simulink model "rubik_cube_solver"  (R2022b)
settings: Solver=FixedStepDiscrete  StartTime=0.0  StopTime=10.0  RelTol=1e-3
InitFcn:
  | mbd_s32k_consistency_checks(bdroot(gcs));
undefined symbols (not defined in the file or in its folder): LQFP
libraries: mbd_s32k1xx_ec_toolbox x5
settings Model: Creator=leona  LastModifiedBy=aless
settings DataIOCC: ExternalInput=off  InitialState=off  SaveOutput=off  SignalLogging=off  SaveTime=off
settings OptimizationCC: DefaultParameterBehavior=Inlined  EnhancedBackFolding=on  PassReuseOutputArgsAs=Individual arguments  ZeroExternalMemoryAtStartup=off  ZeroInternalMemoryAtStartup=off  OptimizeBlockOrder=speed  DifferentSizesBufferReuse=on  OptimizationCustomize=off  EfficientTunableParamExpr=on
settings DebuggingCC: InheritedTsInSrcMsg=none  SingleTaskRateTransMsg=error  ParameterTunabilityLossMsg=error  UnconnectedInputMsg=error  UnconnectedOutputMsg=error  UnconnectedLineMsg=error  UnknownTsInhSupMsg=error
settings HardwareCC: ProdBitPerPointer=32  ProdBitPerSizeT=32  ProdBitPerPtrDiffT=32  ProdLargestAtomicInteger=Long  ProdLargestAtomicFloat=Double  ProdWordSize=32  ProdHWDeviceType=ARM Compatible->ARM Cortex
settings SFSimCC: MATLABDynamicMemAlloc=off
settings RTWCC: Description=Model Based Design Toolbox S32K1xx Code Generation Target  SystemTargetFile=mbd_s32k.tlc  MakeCommand=mbd_s32k_make_rtw COPY_MDLREF_INCLUDES=0  TemplateMakefile=mbd_s32k.tmf
settings CodeAppCC: ForceParamTrailComments=on  IgnoreCustomStorageClasses=off  OperatorAnnotations=on  SimulinkDataObjDesc=on  SFDataObjDesc=on  InsertBlockDesc=on
settings STFCustomTargetCC: TargetLangStandard=C99 (ISO)  MultiwordLength=256  CombineOutputUpdateFcns=on  ERTCustomFileBanners=on  SupportContinuousTime=off  SupportNonInlinedSFcns=off  RemoveResetFunc=on  MATLABClassNameForMDSCustomization=Simulink.SoftwareTarget.ERTCustomization  SystemTargetFile=mbd_s32k.tlc
settings ERTTargetCC: TargetLangStandard=C99 (ISO)  ParMdlRefBuildCompliant=off  CompOptLevelCompliant=off  ConcurrentExecutionCompliant=off  ModelStepFunctionPrototypeControlCompliant=off  CPPClassGenCompliant=off  UseToolchainInfoCompliant=off  InlinedParameterPlacement=NonHierarchical  ERTSrcFileBannerTemplate=mbd_ert_code_template.cgt  ERTHdrFileBannerTemplate=mbd_ert_code_template.cgt  ERTDataSrcFileTemplate=mbd_ert_code_template.cgt  ERTDataHdrFileTemplate=mbd_ert_code_template.cgt  ERTCustomFileTemplate=example_file_process.tlc

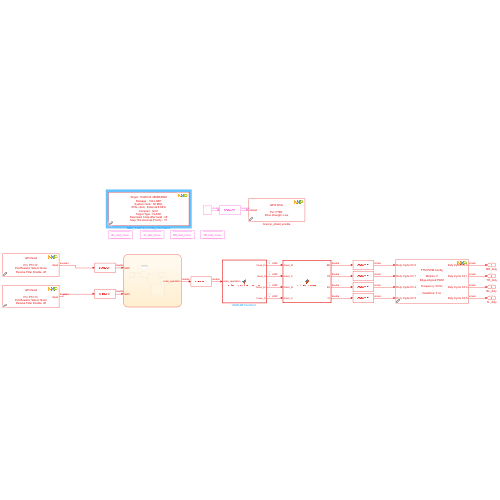
[thumbnail: Simulink's stored preview of the top-level diagram]
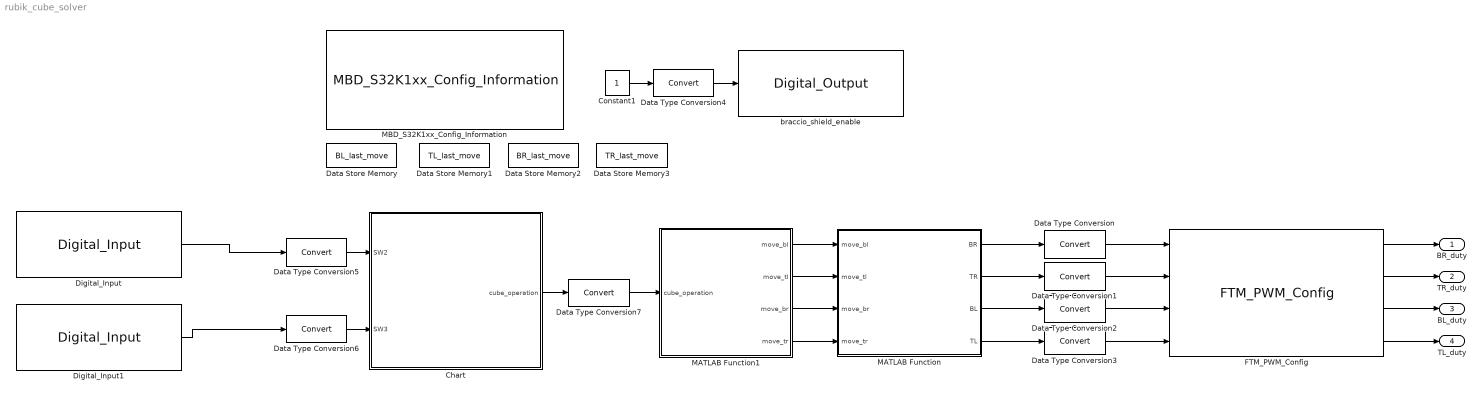
== system rubik_cube_solver ==
  Chart : Stateflow chart  TreatAsAtomicUnit=on
  Constant1 : Constant
  Data Store Memory : DataStoreMemory  DataStoreName=BL_last_move  WriteAfterWriteMsg=warning  ShowAdditionalParam=off
  Data Store Memory1 : DataStoreMemory  DataStoreName=TL_last_move  WriteAfterWriteMsg=warning  ShowAdditionalParam=off
  Data Store Memory2 : DataStoreMemory  DataStoreName=BR_last_move  WriteAfterWriteMsg=warning  ShowAdditionalParam=off
  Data Store Memory3 : DataStoreMemory  DataStoreName=TR_last_move  WriteAfterWriteMsg=warning  ShowAdditionalParam=off
  Data Type Conversion{,1..7} (8 alike) : DataTypeConversion  SaturateOnIntegerOverflow=off  RndMeth=Floor
  Digital_Input : mbd_s32k1xx_ec_toolbox/GPIO Blocks/Digital_Input  gpio_pin=PTC12: [PTC12 | Port C I/O]  pull_resistor=None  passive_filter=off
  Digital_Input1 : mbd_s32k1xx_ec_toolbox/GPIO Blocks/Digital_Input  gpio_pin=PTC13: [PTC13 | Port C I/O]  pull_resistor=None  passive_filter=off
  FTM_PWM_Config : mbd_s32k1xx_ec_toolbox/Motor Control Blocks/FTM Blocks/FTM_PWM_Config  ftmModule=0  ftmMode=Edge-Aligned PWM  ftmSourceClock=80 MHz  swcontrol_enable=off  chan0En=on  chan0Type=Independent  chan2En=off  chan2Type=Independent  chan4En=on  chan4Type=Independent  chan6En=off  chan6Type=Independent  ftmPwmUnits=Hz  outFrequency=50  ftmPeriod=25000  ftmPrescaler=Divide by 64  deadtimeUnits=Nanoseconds  deadtimeNs=0  deadtimeTicks=0  deadtimePrescaler=Divide by 1  dutyCycleCh0=0.03  dutyCycleCh1=0.125  dutyCycleCh2=0.025  dutyCycleCh3=0.025  dutyCycleCh4=0.025  dutyCycleCh5=0.025  dutyCycleCh6=0.25  dutyCycleCh7=0.25  dutyCycleSim=on  startAfterInit=on  showAdvOpt=on  pinFtmCh0=PTD15: [FTM0_CH0 | FTM Channel]  pinFtmCh1=PTD16: [FTM0_CH1 | FTM Channel]  pinPolCh0=Active High  pinPolCh1=Active High  outputComplem0=Main duplicated  outputLevel0=Low  outputLevel1=Low  pinFtmCh2=PTB14: [FTM0_CH2 | FTM Channel]  pinFtmCh3=PTC3: [FTM0_CH3 | FTM Channel]  pinPolCh2=Active High  pinPolCh3=Active High  outputComplem2=Main duplicated  outputLevel2=Low  outputLevel3=Low  pinFtmCh4=PTB4: [FTM0_CH4 | FTM Channel]  pinFtmCh5=PTB5: [FTM0_CH5 | FTM Channel]  pinPolCh4=Active High  pinPolCh5=Active High  outputComplem4=Main duplicated  outputLevel4=Low  outputLevel5=Low  pinFtmCh6=PTE8: [FTM0_CH6 | FTM Channel]  pinFtmCh7=None  pinPolCh6=Active High  pinPolCh7=Active High  outputComplem6=Main duplicated  outputLevel6=Low  outputLevel7=Low  initTrigger=off  chTrigger0=off  chTrigger1=off  chTrigger2=off  chTrigger3=off  chTrigger4=off  chTrigger5=off  chTrigger6=off  chTrigger7=off  mcuTargetUpdate=on  pwmSyncTrg=Software trigger  pwmSyncHwRouting=TRGMUX_FTM7  pwmSyncTrg0=off  pwmSyncTrg1=off  pwmSyncTrg2=off  pwmSyncAutoClear=on  pwmSyncMinLoad=on  pwmSyncMaxLoad=on  pwmSyncInvert=System Clock  pwmSyncOutControl=System Clock  pwmSyncOutMask=System Clock  pwmSyncCounterInitial=System Clock  pwmSyncPoints=Update now  reloadEnable=off  reloadPriority=15  reloadHalfCycle=off  reloadHCR=0  reloadFrequency=0  chnMatch0=off  chnMatch1=off  chnMatch2=off  chnMatch3=off  chnMatch4=off  chnMatch5=off  chnMatch6=off  chnMatch7=off  pwmFaultProtection=off  pwmFaultInterrupt=off  pwmFaultClearing=Fault control disabled  pwmFaultPinState=Safe Value  pwmFaultFilterValue=0  pwmFaultPriority=15  fault_disen_0=off  fault_filter_0=off  fault_polarity_0=Active High  fault_disen_1=off  fault_filter_1=off  fault_polarity_1=Active high  fault_disen_2=off  fault_filter_2=off  fault_polarity_2=Active high  fault_disen_3=off  fault_filter_3=off  fault_polarity_3=Active high  fault_pin_0=None  fault_pin_1=None  fault_pin_2=None  fault_pin_3=None
  MATLAB Function : MATLAB Function  TreatAsAtomicUnit=on
  MATLAB Function1 : MATLAB Function  TreatAsAtomicUnit=on
  MBD_S32K1xx_Config_Information : mbd_s32k1xx_ec_toolbox/MBD_S32K1xx_Config_Information  mbdt_ver=0  disp_str=|  config_params=[]  mcu_target_name=S32K144  mcu_target_package=100-LQFP  mcu_target_sram_size=48KB  mcu_system_clock_freq=80  mcu_xtal_freq=External 8  mcu_steptick_timer=LPIT Channel 0  mcu_steptick_prio=15  ds_import_enable=on  target_compiler=GCC  target_memory=FLASH  gcc_target_compile_opts=-mthumb -mfloat-abi=hard -mfpu=fpv4-sp-d16 -O1 -g -gstrict-dwarf  gcc_target_assemble_opts=-mthumb -mfloat-abi=hard -mfpu=fpv4-sp-d16 -g  gcc_target_link_opts=-mthumb -mfloat-abi=hard -mfpu=fpv4-sp-d16  gcc_target_default_lcf=on  gcc_target_user_lcf=S32K144_48_flash.ld  ghs_target_compile_opts=-cpu=cortexm4f -thumb -fpu=vfpv4_d16 -fsingle -Ogeneral -Wundef -Wimplicit-int -Wshadow -Wtrigraphs --no_commons --gnu_asm -gnu99 -gdwarf-2 -G  ghs_target_assemble_opts=-cpu=cortexm4f -fpu=vfpv4_d16  ghs_target_link_opts=-cpu=cortexm4f -thumb -fpu=vfpv4_d16  ghs_target_default_lcf=on  ghs_target_user_lcf=S32K144_48_flash.ld  iar_target_compile_opts=--cpu=Cortex-M4F --thumb --fpu=VFPv4_sp -Ol -e --debug --dlib_config normal  iar_target_assemble_opts=--cpu Cortex-M4F --thumb --fpu VFPv4_sp  iar_target_link_opts=--no_exceptions --vfe --inline  iar_target_default_lcf=on  iar_target_user_lcf=S32K144_48_flash.icf  pil_download_enable=off  rbl_download_enable=off  rbl_start_delay=5000  rbl_download_interface=OpenSDA  rbl_restart_request=off  rbl_com_port=Custom  rbl_com_port_custom=COM18  pil_download_rate=115200  pil_download_rate_custom=115200  pil_opensda_drive=Custom  pil_opensda_drive_custom=D  jtag_interface=OpenSDA Embedded Debug  jlink_default_path=on  jlink_user_path=C:\Program Files\SEGGER\JLink\  pil_uart_instance=1  pil_uart_rx=PTC6: [LPUART1_RX | Receive]  pil_uart_tx=PTC7: [LPUART1_TX | Transmit]  FTM_PWM_PcrCheckEnDis=on  FTM_Input_Edge_Inputs_PcrCheckEnDis=on  FTM_Dual_Edge_Inputs_PcrCheckEnDis=on  FTM_Quadrature_Inputs_PcrCheckEnDis=on  FTM_Hall_Sensor_Inputs_PcrCheckEnDis=on  LPTMR_PcrCheckEnDis=on  PIT_PcrCheckEnDis=on  RTC_PcrCheckEnDis=on  FlexCAN_PcrCheckEnDis=on  LIN_PcrCheckEnDis=on  FlexIO_PcrCheckEnDis=on  LPI2C_PcrCheckEnDis=on  LPSPI_PcrCheckEnDis=on  LPUART_PcrCheckEnDis=on  CMP_PcrCheckEnDis=on  GPIO_OutputPcrCheckEnDis=on  GPIO_InputPcrCheckEnDis=on  SBC_PcrCheckEnDis=on  BMS_PcrCheckEnDis=on  AMMCLIB_PcrCheckEnDis=on  FM_PcrCheckEnDis=on  Profile_PcrCheckEnDis=on  ConfigParams_PcrCheckEnDis=on  ModelRef_PcrCheckEnDis=on  PDB0_PcrCheckEnDis=on  CSEc_PcrCheckEnDis=on  eDMA_PcrCheckEnDis=on  FLASH_PcrCheckEnDis=on  ADC_PcrCheckEnDis=on  WDOG_PcrCheckEnDis=on
      | Target : S32K144-64KB_SRAM
      | Package : 100-pin
      | System clock : 80 MHz
      | XTAL clock : External 8 MHz
      | Compiler : IAR
      | Target Type : FLASH
      | Download Code after build : off
      | Step Tick Interrupt Priority : 15
  braccio_shield_enable : mbd_s32k1xx_ec_toolbox/GPIO Blocks/Digital_Output  gpio_pin=PTB3: [PTB3 | Port B I/O]  init_val=Low  drive_strength=Low
  BR_duty : Outport
  TR_duty : Outport  Port=2
  BL_duty : Outport  Port=3
  TL_duty : Outport  Port=4
  wires:
  Constant1/1 -> Data Type Conversion4/1
  Data Type Conversion1/1 -> FTM_PWM_Config/2
  Data Type Conversion3/1 -> FTM_PWM_Config/4
  MATLAB Function/2(TR) -> Data Type Conversion1/1
  FTM_PWM_Config/3 -> BL_duty/1
  FTM_PWM_Config/1 -> BR_duty/1
  Data Type Conversion/1 -> FTM_PWM_Config/1
  MATLAB Function1/2(move_tl) -> MATLAB Function/2(move_tl)
  FTM_PWM_Config/2 -> TR_duty/1
  Data Type Conversion2/1 -> FTM_PWM_Config/3
  FTM_PWM_Config/4 -> TL_duty/1
  MATLAB Function1/3(move_br) -> MATLAB Function/3(move_br)
  MATLAB Function1/4(move_tr) -> MATLAB Function/4(move_tr)
  MATLAB Function/4(TL) -> Data Type Conversion3/1
  MATLAB Function/1(BR) -> Data Type Conversion/1
  MATLAB Function/3(BL) -> Data Type Conversion2/1
  Data Type Conversion4/1 -> braccio_shield_enable/1
  MATLAB Function1/1(move_bl) -> MATLAB Function/1(move_bl)
  Data Type Conversion6/1 -> Chart/2(SW3)
  Data Type Conversion5/1 -> Chart/1(SW2)
  Digital_Input/1 -> Data Type Conversion5/1
  Digital_Input1/1 -> Data Type Conversion6/1
  Chart/1(cube_operation) -> Data Type Conversion7/1
  Data Type Conversion7/1 -> MATLAB Function1/1(cube_operation)

== matlab function rubik_cube_solver/MATLAB Function1 ==
  data: cube_operation input; move_bl output; move_tl output; move_br output; move_tr output
function [move_bl, move_tl, move_br, move_tr] = cube_operation_decoder(cube_operation)
% This function takes as input the code for a cube operation and converts
% it as positions of the 4 servo motors. The operations must be a 4 digit
% unsigned integer, encoded as follows:
%   - first digit [0, 1]: open/close left grip;
%   - second digit [0, 1]: open/close right grip;
%   - third digit [0, 1, 2]: set left arm to 90/0/180 degrees
%   - fourth digit [0, 1, 2]: set right arm to 90/0/180 degress

x1 = int32(mod(cube_operation/1000, 10));
x2 = int32(mod(cube_operation/100, 10));
x3 = int32(mod(cube_operation/10, 10));
x4 = int32(mod(cube_operation, 10));

move_tl = x1;
move_tr = x2;
move_bl = x3;
move_br = x4;

== matlab function rubik_cube_solver/MATLAB Function ==
  data: BR output; TR output; move_bl input; BL output; move_tl input; move_br input; move_tr input; TL output
function [BR, TR, BL, TL] = actuate_servos(move_bl, move_tl, move_br, move_tr)
% This function takes as input as specific number associated to a movement
% of the 4 servo motors (BL = Bottom Left, TL = Top Left, BR = Bottom Right,
% TR = Top Right) and it gives as output the 4 relative duty cycles needed to
% obtain that movement. 

min_duty = 0.025;
max_duty = 0.125;

duty_0_deg = min_duty;
duty_grip_open = min_duty + (max_duty-min_duty)/3;
duty_grip_closed = min_duty + (max_duty-min_duty)/15; 
duty_90_deg = min_duty + (max_duty-min_duty)/2;
duty_180_deg = max_duty;

switch (move_tl)
    case 0                  % Open left grip
        TL = duty_grip_open;
    case 1                  % Close left grip
        TL = duty_grip_closed;
    otherwise               % Open left grip
        TL = duty_grip_open;
end

switch (move_tr)
    case 0                  % Open right grip
        TR = duty_grip_open;
    case 1                  % Close right grip
        TR = duty_grip_closed;
    otherwise               % Open right grip
        TR = duty_grip_open;
end

switch (move_bl)
    case 0                  % Left arm straight
        BL = duty_90_deg;
    case 1                  % Left arm at 90° clockwise
        BL = duty_0_deg;
    case 2                 % Left arm at 90° counter-clockwise
        BL = duty_180_deg;
    otherwise
        BL = duty_90_deg;
end

switch (move_br)
    case 0                  % Right arm straight
        BR = duty_90_deg;
    case 1                  % Right arm at 90° clockwise
        BR = duty_0_deg;
    case 2                 % Right arm at 90° counter-clockwise
        BR = duty_180_deg;
    otherwise
        BR = duty_90_deg;
end

% Update current position of the motors
BL_last_move = move_bl;
TL_last_move = move_tl;
BR_last_move = move_br;
TR_last_move = move_tr;

== stateflow chart rubik_cube_solver/Chart ==
  state Li [commented out]
    en:
    %LTpp
    %RMm
    state fase1 [commented out]
      en:
      cube_operation=0100;
    state fase1bis [commented out]
      en:
      cube_operation=0110;
    state fase2 [commented out]
      en:
      cube_operation=1110;
    state fase4 [commented out]
      en:
      cube_operation=1120;
    state fase3bis [commented out]
      en:
      cube_operation=1020;
    state fase3 [commented out]
      en:
      cube_operation=1010;
    state fase5bis [commented out]
      en:
      cube_operation=0100;
    state fase6 [commented out]
      en:
      cube_operation=1100
    state fase5 [commented out]
      en:
      cube_operation=0120;
    state fase8bis [commented out]
      en:
      cube_operation=1000;
    state fase8 [commented out]
      en:
      cube_operation=1001;
    state fase7 %RMm [commented out]
      en:
      cube_operation=1101;
    state fase9 [commented out]
      en:
      cube_operation=1100;
    (default) -> Li.fase1 [commented out]
    Li.fase1 -> Li.fase1bis [commented out] : [after(delay_ms,msec)]
    Li.fase1bis -> Li.fase2 [commented out] : [after(delay_ms,msec)]
    Li.fase2 -> Li.fase3 [commented out] : [after(delay_ms,msec)]
    Li.fase3bis -> Li.fase4 [commented out] : [after(delay_ms,msec)]
    Li.fase3 -> Li.fase3bis [commented out] : [after(delay_ms,msec)]
    Li.fase4 -> Li.fase5 [commented out] : [after(delay_ms,msec)]
    Li.fase5bis -> Li.fase6 [commented out] : [after(delay_ms,msec)]
    Li.fase5 -> Li.fase5bis [commented out] : [after(delay_ms,msec)]
    Li.fase6 -> fase7 %RMm [commented out] : [after(delay_ms,msec)]
    fase7 %RMm -> Li.fase8 [commented out] : [after(delay_ms,msec)]
    Li.fase8 -> fase8bis [commented out] : [after(delay_ms,msec)]
    fase8bis -> Li.fase9 [commented out] : [after(delay_ms,msec)]
  state L [commented out]
    en:
    %LTpp
    %RMp
    state fase1 [commented out]
      en:
      cube_operation=0100;
    state fase1bis [commented out]
      en:
      cube_operation=0110;
    state fase2 [commented out]
      en:
      cube_operation=1110;
    state fase4 [commented out]
      en:
      cube_operation=1120;
    state fase3bis [commented out]
      en:
      cube_operation=1020;
    state fase3 [commented out]
      en:
      cube_operation=1010;
    state fase5bis [commented out]
      en:
      cube_operation=0100;
    state fase6 [commented out]
      en:
      cube_operation=1100
    state fase5 [commented out]
      en:
      cube_operation=0120;
    state fase8 [commented out]
      en:
      cube_operation=1101;
    state fase7bis [commented out]
      en:
      cube_operation=1001;
    state fase7 %RMp [commented out]
      en:
      cube_operation=1000;
    state fase9 [commented out]
      en:
      cube_operation=1100;
    L.fase1 -> L.fase1bis [commented out] : [after(delay_ms,msec)]
    L.fase1bis -> L.fase2 [commented out] : [after(delay_ms,msec)]
    L.fase2 -> L.fase3 [commented out] : [after(delay_ms,msec)]
    L.fase3bis -> L.fase4 [commented out] : [after(delay_ms,msec)]
    L.fase3 -> L.fase3bis [commented out] : [after(delay_ms,msec)]
    L.fase4 -> L.fase5 [commented out] : [after(delay_ms,msec)]
    L.fase5bis -> L.fase6 [commented out] : [after(delay_ms,msec)]
    L.fase5 -> L.fase5bis [commented out] : [after(delay_ms,msec)]
    L.fase6 -> fase7 %RMp [commented out] : [after(delay_ms,msec)]
    fase7 %RMp -> L.fase7bis [commented out] : [after(delay_ms,msec)]
    L.fase7bis -> L.fase8 [commented out] : [after(delay_ms,msec)]
    L.fase8 -> L.fase9 [commented out] : [after(delay_ms,msec)]
  state L2 [commented out]
    en:
    %LTpp
    %RMpp
    state fase1 [commented out]
      en:
      cube_operation=0100;
    state fase1bis [commented out]
      en:
      cube_operation=0110;
    state fase2 [commented out]
      en:
      cube_operation=1110;
    state fase4 [commented out]
      en:
      cube_operation=1120;
    state fase3bis [commented out]
      en:
      cube_operation=1020;
    state fase3 [commented out]
      en:
      cube_operation=1010;
    state fase5bis [commented out]
      en:
      cube_operation=0100;
    state fase6 [commented out]
      en:
      cube_operation=1100
    state fase5 [commented out]
      en:
      cube_operation=0120;
    state fase12 %RMpp [commented out]
      en:
      cube_operation=1000;
    state fase7bis [commented out]
      en:
      cube_operation=1001;
    state fase9 [commented out]
      en:
      cube_operation=1102;
    state fase8 [commented out]
      en:
      cube_operation=1101;
    state fase10 [commented out]
      en:
      cube_operation=1002;
    state fase11 [commented out]
      en:
      cube_operation=1100;
    state fase10bis [commented out]
      en:
      cube_operation=1000;
    L2.fase1 -> L2.fase1bis [commented out] : [after(delay_ms,msec)]
    L2.fase1bis -> L2.fase2 [commented out] : [after(delay_ms,msec)]
    L2.fase2 -> L2.fase3 [commented out] : [after(delay_ms,msec)]
    L2.fase3bis -> L2.fase4 [commented out] : [after(delay_ms,msec)]
    L2.fase3 -> L2.fase3bis [commented out] : [after(delay_ms,msec)]
    L2.fase4 -> L2.fase5 [commented out] : [after(delay_ms,msec)]
    L2.fase5bis -> L2.fase6 [commented out] : [after(delay_ms,msec)]
    L2.fase5 -> L2.fase5bis [commented out] : [after(delay_ms,msec)]
    L2.fase6 -> fase12 %RMpp [commented out] : [after(delay_ms,msec)]
    fase12 %RMpp -> L2.fase7bis [commented out] : [after(delay_ms,msec)]
    L2.fase7bis -> L2.fase8 [commented out] : [after(delay_ms,msec)]
    L2.fase9 -> L2.fase10 [commented out] : [after(delay_ms,msec)]
    L2.fase8 -> L2.fase9 [commented out] : [after(delay_ms,msec)]
    L2.fase10 -> fase10bis [commented out] : [after(delay_ms,msec)]
    fase10bis -> L2.fase11 [commented out] : [after(delay_ms,msec)]
  state U [commented out]
    %RTpp
    %LMp
    state fase1 %RTpp [commented out]
      en:
      cube_operation=1000;
    state fase2 [commented out]
      en:
      cube_operation=1001;
    state fase3 [commented out]
      en:
      cube_operation=1101;
    state fase6 [commented out]
      en:
      cube_operation=1102;
    state fase5 [commented out]
      en:
      cube_operation=0102;
    state fase4 [commented out]
      en:
      cube_operation=0101;
    state fase8 [commented out]
      en:
      cube_operation=1000;
    state fase9 [commented out]
      en:
      cube_operation=1100;
    state fase7 [commented out]
      en:
      cube_operation=1002;
    state fase12 [commented out]
      en:
      cube_operation=1110;
    state fase11 [commented out]
      en:
      cube_operation=0110;
    state fase10 %LMp [commented out]
      en:
      cube_operation=0100;
    state fase13 [commented out]
      en:
      cube_operation=1100;
    (default) -> U.fase1 %RTpp [commented out]
    U.fase2 -> U.fase3 [commented out] : [after(delay_ms,msec)]
    U.fase1 %RTpp -> U.fase2 [commented out] : [after(delay_ms,msec)]
    U.fase3 -> U.fase4 [commented out] : [after(delay_ms,msec)]
    U.fase4 -> U.fase5 [commented out] : [after(delay_ms,msec)]
    U.fase5 -> U.fase6 [commented out] : [after(delay_ms,msec)]
    U.fase6 -> U.fase7 [commented out] : [after(delay_ms,msec)]
    U.fase7 -> U.fase8 [commented out] : [after(delay_ms,msec)]
    U.fase8 -> U.fase9 [commented out] : [after(delay_ms,msec)]
    U.fase9 -> fase10 %LMp [commented out] : [after(delay_ms,msec)]
    U.fase11 -> U.fase12 [commented out] : [after(delay_ms,msec)]
    fase10 %LMp -> U.fase11 [commented out] : [after(delay_ms,msec)]
    U.fase12 -> U.fase13 [commented out] : [after(delay_ms,msec)]
  state U2 [commented out]
    %RTpp
    %LMpp
    state fase1 %RTpp [commented out]
      en:
      cube_operation=1000;
    state fase2 [commented out]
      en:
      cube_operation=1001;
    state fase3 [commented out]
      en:
      cube_operation=1101;
    state fase6 [commented out]
      en:
      cube_operation=1102;
    state fase5 [commented out]
      en:
      cube_operation=0102;
    state fase4 [commented out]
      en:
      cube_operation=0101;
    state fase8 [commented out]
      en:
      cube_operation=1000;
    state fase9 [commented out]
      en:
      cube_operation=1100;
    state fase7 [commented out]
      en:
      cube_operation=1002;
    state fase11 [commented out]
      en:
      cube_operation=0110;
    state fase10 %LMpp [commented out]
      en:
      cube_operation=0100;
    state fase12 [commented out]
      en:
      cube_operation=1110;
    state fase13 [commented out]
      en:
      cube_operation=1120;
    state fase14 [commented out]
      en:
      cube_operation=0120;
    state fase15 [commented out]
      en:
      cube_operation=0100;
    state fase16 [commented out]
      en:
      cube_operation=1100;
    (default) -> U2.fase1 %RTpp [commented out]
    U2.fase2 -> U2.fase3 [commented out] : [after(delay_ms,msec)]
    U2.fase1 %RTpp -> U2.fase2 [commented out] : [after(delay_ms,msec)]
    U2.fase3 -> U2.fase4 [commented out] : [after(delay_ms,msec)]
    U2.fase4 -> U2.fase5 [commented out] : [after(delay_ms,msec)]
    U2.fase5 -> U2.fase6 [commented out] : [after(delay_ms,msec)]
    U2.fase6 -> U2.fase7 [commented out] : [after(delay_ms,msec)]
    U2.fase7 -> U2.fase8 [commented out] : [after(delay_ms,msec)]
    U2.fase8 -> U2.fase9 [commented out] : [after(delay_ms,msec)]
    U2.fase9 -> fase10 %LMpp [commented out] : [after(delay_ms,msec)]
    U2.fase11 -> U2.fase12 [commented out] : [after(delay_ms,msec)]
    fase10 %LMpp -> U2.fase11 [commented out] : [after(delay_ms,msec)]
    U2.fase12 -> U2.fase13 [commented out] : [after(delay_ms,msec)]
    U2.fase13 -> fase14 [commented out] : [after(delay_ms,msec)]
    fase14 -> fase15 [commented out] : [after(delay_ms,msec)]
    fase15 -> fase16 [commented out] : [after(delay_ms,msec)]
  state waiting_for_cube
    en:
    %R = randi([1, 6], 3, 3, 6);
    solution = string(repmat(' ', 1, 45))
    %sol=Solve45(rubgen(3,23))
    sequence
    du:
    cube_operation=0100;
    SW2_status=SW2;
    end
  state waiting_to_start
    en:
    du:
    cube_operation=1100;
    SW2_status=SW2;
    SW3_status=SW3;
  state cube_reading
    en:
  state cube_solving
    en:
  state Ui [commented out]
    %RTpp
    %LMm
    state fase1 %RTpp [commented out]
      en:
      cube_operation=1000;
    state fase2 [commented out]
      en:
      cube_operation=1001;
    state fase3 [commented out]
      en:
      cube_operation=1101;
    state fase6 [commented out]
      en:
      cube_operation=1102;
    state fase5 [commented out]
      en:
      cube_operation=0102;
    state fase4 [commented out]
      en:
      cube_operation=0101;
    state fase8 [commented out]
      en:
      cube_operation=1000;
    state fase9 [commented out]
      en:
      cube_operation=1100;
    state fase7 [commented out]
      en:
      cube_operation=1002;
    state fase12 [commented out]
      en:
      cube_operation=0100;
    state fase11 [commented out]
      en:
      cube_operation=0110;
    state fase10 %LMm [commented out]
      en:
      cube_operation=1110;
    state fase13 [commented out]
      en:
      cube_operation=1100;
    (default) -> Ui.fase1 %RTpp [commented out]
    Ui.fase2 -> Ui.fase3 [commented out] : [after(delay_ms,msec)]
    Ui.fase1 %RTpp -> Ui.fase2 [commented out] : [after(delay_ms,msec)]
    Ui.fase3 -> Ui.fase4 [commented out] : [after(delay_ms,msec)]
    Ui.fase4 -> Ui.fase5 [commented out] : [after(delay_ms,msec)]
    Ui.fase5 -> Ui.fase6 [commented out] : [after(delay_ms,msec)]
    Ui.fase6 -> Ui.fase7 [commented out] : [after(delay_ms,msec)]
    Ui.fase7 -> Ui.fase8 [commented out] : [after(delay_ms,msec)]
    Ui.fase8 -> Ui.fase9 [commented out] : [after(delay_ms,msec)]
    Ui.fase9 -> fase10 %LMm [commented out] : [after(delay_ms,msec)]
    Ui.fase11 -> Ui.fase12 [commented out] : [after(delay_ms,msec)]
    fase10 %LMm -> Ui.fase11 [commented out] : [after(delay_ms,msec)]
    Ui.fase12 -> Ui.fase13 [commented out] : [after(delay_ms,msec)]
  state F [commented out]
    en:
    %RTm
    %LMp
    state fase1 [commented out]
      en:
      cube_operation=0100;
    state fase2 [commented out]
      en:
      cube_operation=0101;
    state fase3 [commented out]
      en:
      cube_operation=1101;
    state fase6 [commented out]
      en:
      cube_operation=1100
    state fase5 [commented out]
      en:
      cube_operation=1000;
    state fase4 [commented out]
      en:
      cube_operation=1001;
    state fase7 %LMp [commented out]
      en:
      cube_operation=0100;
    state fase8 [commented out]
      en:
      cube_operation=0110;
    state fase9 [commented out]
      en:
      cube_operation=1110;
    state fase10 [commented out]
      en:
      cube_operation=1100;
    (default) -> F.fase1 [commented out]
    F.fase2 -> F.fase3 [commented out] : [after(delay_ms,msec)]
    F.fase1 -> F.fase2 [commented out] : [after(delay_ms,msec)]
    F.fase3 -> F.fase4 [commented out] : [after(delay_ms,msec)]
    F.fase5 -> F.fase6 [commented out] : [after(delay_ms,msec)]
    F.fase4 -> F.fase5 [commented out] : [after(delay_ms,msec)]
    F.fase6 -> F.fase7 %LMp [commented out] : [after(delay_ms,msec)]
    F.fase7 %LMp -> F.fase8 [commented out] : [after(delay_ms,msec)]
    F.fase9 -> F.fase10 [commented out] : [after(delay_ms,msec)]
    F.fase8 -> F.fase9 [commented out] : [after(delay_ms,msec)]
  state Di [commented out]
    en:
    %LMm
    state fase1 %LMm [commented out]
      en:
      cube_operation=1110;
    state fase2 [commented out]
      en:
      cube_operation=0110;
    state fase3 [commented out]
      en:
      cube_operation=0100;
    state fase4 [commented out]
      en:
      cube_operation=1100;
    (default) -> fase1 %LMm [commented out]
    fase1 %LMm -> Di.fase2 [commented out] : [after(delay_ms,msec)]
    Di.fase2 -> Di.fase3 [commented out] : [after(delay_ms,msec)]
    Di.fase3 -> Di.fase4 [commented out] : [after(delay_ms,msec)]
  state R [commented out]
    en:
    %RMp
    state fase1 %RMp [commented out]
      en:
      cube_operation=1000;
    state fase2 [commented out]
      en:
      cube_operation=1001;
    state fase3 [commented out]
      en:
      cube_operation=1101;
    state fase4 [commented out]
      en:
      cube_operation=1100;
    (default) -> fase1 %RMp [commented out]
    fase1 %RMp -> R.fase2 [commented out] : [after(delay_ms,msec)]
    R.fase2 -> R.fase3 [commented out] : [after(delay_ms,msec)]
    R.fase3 -> R.fase4 [commented out] : [after(delay_ms,msec)]
  state R2 [commented out]
    en:
    %RMpp
    state fase1 %RMpp [commented out]
      en:
      cube_operation=1000;
    state fase2 [commented out]
      en:
      cube_operation=1001;
    state fase4 [commented out]
      en:
      cube_operation=1102;
    state fase3 [commented out]
      en:
      cube_operation=1101;
    state fase5 [commented out]
      en:
      cube_operation=1002;
    state fase6 [commented out]
      en:
      cube_operation=1000;
    state fase7 [commented out]
      en:
      cube_operation=1100;
    (default) -> fase1 %RMpp [commented out]
    fase1 %RMpp -> R2.fase2 [commented out] : [after(delay_ms,msec)]
    R2.fase2 -> R2.fase3 [commented out] : [after(delay_ms,msec)]
    R2.fase3 -> R2.fase4 [commented out] : [after(delay_ms,msec)]
    R2.fase4 -> R2.fase5 [commented out] : [after(delay_ms,msec)]
    R2.fase5 -> R2.fase6 [commented out] : [after(delay_ms,msec)]
    R2.fase6 -> R2.fase7 [commented out] : [after(delay_ms,msec)]
  state D [commented out]
    en:
    %LMp
    state fase1 %LMp [commented out]
      en:
      cube_operation=0100;
    state fase2 [commented out]
      en:
      cube_operation=0110;
    state fase3 [commented out]
      en:
      cube_operation=1110;
    state fase4 [commented out]
      en:
      cube_operation=1100;
    (default) -> fase1 %LMp [commented out]
    fase1 %LMp -> D.fase2 [commented out] : [after(delay_ms,msec)]
    D.fase2 -> D.fase3 [commented out] : [after(delay_ms,msec)]
    D.fase3 -> D.fase4 [commented out] : [after(delay_ms,msec)]
  state D2 [commented out]
    en:
    %LMpp
    state fase1 %LMpp [commented out]
      en:
      cube_operation=0100;
    state fase2 [commented out]
      en:
      cube_operation=0110;
    state fase4 [commented out]
      en:
      cube_operation=1120;
    state fase3 [commented out]
      en:
      cube_operation=1110;
    state fase6 [commented out]
      en:
      cube_operation=0100;
    state fase5 [commented out]
      en:
      cube_operation=0120;
    state fase7 [commented out]
      en:
      cube_operation=1100;
    (default) -> fase1 %LMpp [commented out]
    fase1 %LMpp -> D2.fase2 [commented out] : [after(delay_ms,msec)]
    D2.fase2 -> D2.fase3 [commented out] : [after(delay_ms,msec)]
    D2.fase3 -> D2.fase4 [commented out] : [after(delay_ms,msec)]
    D2.fase4 -> D2.fase5 [commented out] : [after(delay_ms,msec)]
    D2.fase5 -> D2.fase6 [commented out] : [after(delay_ms,msec)]
    D2.fase6 -> D2.fase7 [commented out] : [after(delay_ms,msec)]
  state Ri [commented out]
    en:
    %RMm
    state fase1 %RMm [commented out]
      en:
      cube_operation=1101;
    state fase2 [commented out]
      en:
      cube_operation=1001;
    state fase3 [commented out]
      en:
      cube_operation=1000;
    state fase4 [commented out]
      en:
      cube_operation=1100;
    (default) -> fase1 %RMm [commented out]
    fase1 %RMm -> Ri.fase2 [commented out] : [after(delay_ms,msec)]
    Ri.fase2 -> Ri.fase3 [commented out] : [after(delay_ms,msec)]
    Ri.fase3 -> Ri.fase4 [commented out] : [after(delay_ms,msec)]
  state F2 [commented out]
    en:
    %RTm
    %LMpp
    state fase1 [commented out]
      en:
      cube_operation=0100;
    state fase2 [commented out]
      en:
      cube_operation=0101;
    state fase3 [commented out]
      en:
      cube_operation=1101;
    state fase4 [commented out]
      en:
      cube_operation=1001;
    state fase7 %LMpp [commented out]
      en:
      cube_operation=0100;
    state fase6 [commented out]
      en:
      cube_operation=1100
    state fase8 [commented out]
      en:
      cube_operation=0110;
    state fase5 [commented out]
      en:
      cube_operation=1000;
    state fase9 [commented out]
      en:
      cube_operation=1110;
    state fase10 [commented out]
      en:
      cube_operation=1120;
    state fase11 [commented out]
      en:
      cube_operation=0120;
    state fase12 [commented out]
      en:
      cube_operation=0100;
    state fase13 [commented out]
      en:
      cube_operation=1100;
    F2.fase2 -> F2.fase3 [commented out] : [after(delay_ms,msec)]
    F2.fase1 -> F2.fase2 [commented out] : [after(delay_ms,msec)]
    F2.fase3 -> F2.fase4 [commented out] : [after(delay_ms,msec)]
    (default) -> F2.fase1 [commented out]
    F2.fase4 -> F2.fase5 [commented out] : [after(delay_ms,msec)]
    F2.fase7 %LMpp -> F2.fase8 [commented out] : [after(delay_ms,msec)]
    F2.fase6 -> F2.fase7 %LMpp [commented out] : [after(delay_ms,msec)]
    F2.fase5 -> F2.fase6 [commented out] : [after(delay_ms,msec)]
    F2.fase8 -> F2.fase9 [commented out] : [after(delay_ms,msec)]
    F2.fase10 -> F2.fase11 [commented out] : [after(delay_ms,msec)]
    F2.fase9 -> F2.fase10 [commented out] : [after(delay_ms,msec)]
    F2.fase11 -> F2.fase12 [commented out] : [after(delay_ms,msec)]
    F2.fase12 -> F2.fase13 [commented out] : [after(delay_ms,msec)]
  state Fi [commented out]
    en:
    %RTm
    %LMm
    state fase1 [commented out]
      en:
      cube_operation=0100;
    state fase2 [commented out]
      en:
      cube_operation=0101;
    state fase3 [commented out]
      en:
      cube_operation=1101;
    state fase4 [commented out]
      en:
      cube_operation=1001;
    state fase6 [commented out]
      en:
      cube_operation=1100
    state fase8 [commented out]
      en:
      cube_operation=0110;
    state fase5 [commented out]
      en:
      cube_operation=1000;
    state fase7 %LMm [commented out]
      en:
      cube_operation=1110;
    state fase9 [commented out]
      en:
      cube_operation=0100;
    state fase10 [commented out]
      en:
      cube_operation=1100;
    Fi.fase2 -> Fi.fase3 [commented out] : [after(delay_ms,msec)]
    Fi.fase1 -> Fi.fase2 [commented out] : [after(delay_ms,msec)]
    Fi.fase3 -> Fi.fase4 [commented out] : [after(delay_ms,msec)]
    (default) -> Fi.fase1 [commented out]
    Fi.fase4 -> Fi.fase5 [commented out] : [after(delay_ms,msec)]
    Fi.fase5 -> Fi.fase6 [commented out] : [after(delay_ms,msec)]
    Fi.fase6 -> Fi.fase7 %LMm [commented out] : [after(delay_ms,msec)]
    Fi.fase7 %LMm -> Fi.fase8 [commented out] : [after(delay_ms,msec)]
    Fi.fase8 -> Fi.fase9 [commented out] : [after(delay_ms,msec)]
    Fi.fase9 -> Fi.fase10 [commented out] : [after(delay_ms,msec)]
  state B [commented out]
    en:
    %RTp
    %LMp
    state fase1 [commented out]
      en:
      cube_operation=1000;
    state fase2 [commented out]
      en:
      cube_operation=1001;
    state fase3 [commented out]
      en:
      cube_operation=1101;
    state fase6 [commented out]
      en:
      cube_operation=1100
    state fase5 [commented out]
      en:
      cube_operation=0100;
    state fase4 [commented out]
      en:
      cube_operation=0101;
    state fase7 %LMp [commented out]
      en:
      cube_operation=0100;
    state fase8 [commented out]
      en:
      cube_operation=0110;
    state fase9 [commented out]
      en:
      cube_operation=1110;
    state fase10 [commented out]
      en:
      cube_operation=1100;
    (default) -> B.fase1 [commented out]
    B.fase2 -> B.fase3 [commented out] : [after(delay_ms,msec)]
    B.fase1 -> B.fase2 [commented out] : [after(delay_ms,msec)]
    B.fase3 -> B.fase4 [commented out] : [after(delay_ms,msec)]
    B.fase5 -> B.fase6 [commented out] : [after(delay_ms,msec)]
    B.fase4 -> B.fase5 [commented out] : [after(delay_ms,msec)]
    B.fase6 -> B.fase7 %LMp [commented out] : [after(delay_ms,msec)]
    B.fase7 %LMp -> B.fase8 [commented out] : [after(delay_ms,msec)]
    B.fase9 -> B.fase10 [commented out] : [after(delay_ms,msec)]
    B.fase8 -> B.fase9 [commented out] : [after(delay_ms,msec)]
  state B2 [commented out]
    en:
    %RTp
    %LMpp
    state fase1 [commented out]
      en:
      cube_operation=1000;
    state fase2 [commented out]
      en:
      cube_operation=1001;
    state fase3 [commented out]
      en:
      cube_operation=1101;
    state fase4 [commented out]
      en:
      cube_operation=0101;
    state fase7 %LMpp [commented out]
      en:
      cube_operation=0100;
    state fase6 [commented out]
      en:
      cube_operation=1100
    state fase8 [commented out]
      en:
      cube_operation=0110;
    state fase5 [commented out]
      en:
      cube_operation=0100;
    state fase9 [commented out]
      en:
      cube_operation=1110;
    state fase10 [commented out]
      en:
      cube_operation=1120;
    state fase11 [commented out]
      en:
      cube_operation=0120;
    state fase12 [commented out]
      en:
      cube_operation=0100;
    state fase13 [commented out]
      en:
      cube_operation=1100;
    B2.fase2 -> B2.fase3 [commented out] : [after(delay_ms,msec)]
    B2.fase1 -> B2.fase2 [commented out] : [after(delay_ms,msec)]
    B2.fase3 -> B2.fase4 [commented out] : [after(delay_ms,msec)]
    (default) -> B2.fase1 [commented out]
    B2.fase4 -> B2.fase5 [commented out] : [after(delay_ms,msec)]
    B2.fase7 %LMpp -> B2.fase8 [commented out] : [after(delay_ms,msec)]
    B2.fase6 -> B2.fase7 %LMpp [commented out] : [after(delay_ms,msec)]
    B2.fase5 -> B2.fase6 [commented out] : [after(delay_ms,msec)]
    B2.fase8 -> B2.fase9 [commented out] : [after(delay_ms,msec)]
    B2.fase10 -> B2.fase11 [commented out] : [after(delay_ms,msec)]
    B2.fase9 -> B2.fase10 [commented out] : [after(delay_ms,msec)]
    B2.fase11 -> B2.fase12 [commented out] : [after(delay_ms,msec)]
    B2.fase12 -> B2.fase13 [commented out] : [after(delay_ms,msec)]
  state Bi [commented out]
    en:
    %RTp
    %LMm
    state fase1 [commented out]
      en:
      cube_operation=1000;
    state fase2 [commented out]
      en:
      cube_operation=1001;
    state fase3 [commented out]
      en:
      cube_operation=1101;
    state fase4 [commented out]
      en:
      cube_operation=0101;
    state fase6 [commented out]
      en:
      cube_operation=1100
    state fase8 [commented out]
      en:
      cube_operation=0110;
    state fase7 %LMm [commented out]
      en:
      cube_operation=1110;
    state fase5 [commented out]
      en:
      cube_operation=0100;
    state fase9 [commented out]
      en:
      cube_operation=0100;
    state fase10 [commented out]
      en:
      cube_operation=1100;
    Bi.fase2 -> Bi.fase3 [commented out] : [after(delay_ms,msec)]
    Bi.fase1 -> Bi.fase2 [commented out] : [after(delay_ms,msec)]
    Bi.fase3 -> Bi.fase4 [commented out] : [after(delay_ms,msec)]
    (default) -> Bi.fase1 [commented out]
    Bi.fase4 -> Bi.fase5 [commented out] : [after(delay_ms,msec)]
    Bi.fase6 -> Bi.fase7 %LMm [commented out] : [after(delay_ms,msec)]
    Bi.fase5 -> Bi.fase6 [commented out] : [after(delay_ms,msec)]
    Bi.fase7 %LMm -> Bi.fase8 [commented out] : [after(delay_ms,msec)]
    Bi.fase8 -> Bi.fase9 [commented out] : [after(delay_ms,msec)]
    Bi.fase9 -> Bi.fase10 [commented out] : [after(delay_ms,msec)]
  (default) -> waiting_for_cube
  waiting_for_cube -> waiting_to_start : [SW2==1 && SW2_status==0]
  waiting_to_start -> cube_reading [order 2] : [SW3==1 && SW3_status==0]
  waiting_to_start -> waiting_for_cube [order 1] : [SW2==1 && SW2_status==0]
  cube_reading -> cube_solving : [after(100,msec)]
  cube_solving -> waiting_to_start : [after(100,msec)]
  data: SW2 input; cube_operation output; SW3 input; SW3_status local =0; SW2_status local double =0; delay_ms constant double =2000; solution local
  function sequence:
    | function sequence
    | solution= Solve45(rubgen(3,23))
    | end
